simulink model "MotorCtrl_DTC_Math"  (R2023b)
settings: Solver=FixedStepDiscrete  StartTime=0.0  StopTime=5  FixedStep=MC_Sim_BaseStep  RelTol=1e-3  EnableMultiTasking=on
values from neighbouring files (symbols this model uses):
  MC_ADC_BitNum = 0.0    [MotorControlDataDictionary_Math.sldd]
  MC_ADC_Offset = 0.0    [MotorControlDataDictionary_Math.sldd]
  MC_ADC_VRef = 1.0    [MotorControlDataDictionary_Math.sldd]
  MC_Const_DutyL = 0.2    [MotorControlDataDictionary_Math.sldd]
  MC_Const_DutyS = 0.8    [MotorControlDataDictionary_Math.sldd]
  MC_CSA_Gain = 1.0    [MotorControlDataDictionary_Math.sldd]
  MC_Input_Vdc = 13.5    [MotorControlDataDictionary_Math.sldd]
  MC_MOS_DeadTime = 1.0E-6    [MotorControlDataDictionary_Math.sldd]
  MC_Motor_Mechinal_Damp = 1.0E-5    [MotorControlDataDictionary_Math.sldd]
  MC_Motor_Mechinal_Fric = 0.0    [MotorControlDataDictionary_Math.sldd]
  MC_Motor_Mechinal_Inertia = 0.0103    [MotorControlDataDictionary_Math.sldd]
  MC_Motor_Phi = 0.0059190254913385806    [MotorControlDataDictionary_Math.sldd]
  MC_Motor_Rotor_Pn = 4.0    [MotorControlDataDictionary_Math.sldd]
  MC_Motor_Stator_Ld = 5.6345E-5    [MotorControlDataDictionary_Math.sldd]
  MC_Motor_Stator_Lq = 5.6345E-5    [MotorControlDataDictionary_Math.sldd]
  MC_Motor_Stator_Rs = 0.0286    [MotorControlDataDictionary_Math.sldd]
  MC_Param_CurrentPI_Ki = 0.0071879639914134473    [MotorControlDataDictionary_Math.sldd]
  MC_Param_CurrentPI_Kp = 0.283220860906427    [MotorControlDataDictionary_Math.sldd]
  MC_Param_CurrentPI_UdInteMax = 7.794228634059948    [MotorControlDataDictionary_Math.sldd]
  MC_Param_CurrentPI_UdInteMin = -7.794228634059948    [MotorControlDataDictionary_Math.sldd]
  MC_Param_CurrentPI_UdMax = 7.794228634059948    [MotorControlDataDictionary_Math.sldd]
  MC_Param_CurrentPI_UdMin = -7.794228634059948    [MotorControlDataDictionary_Math.sldd]
  MC_Param_CurrentPI_UqInteMax = 7.794228634059948    [MotorControlDataDictionary_Math.sldd]
  MC_Param_CurrentPI_UqInteMin = -7.794228634059948    [MotorControlDataDictionary_Math.sldd]
  MC_Param_CurrentPI_UqMax = 7.794228634059948    [MotorControlDataDictionary_Math.sldd]
  MC_Param_CurrentPI_UqMin = -7.794228634059948    [MotorControlDataDictionary_Math.sldd]
  MC_Param_Flux_Gamma = 750000.0    [MotorControlDataDictionary_Math.sldd]
  MC_Param_Flux_Lalpha = 5.6345E-5    [MotorControlDataDictionary_Math.sldd]
  MC_Param_Flux_Lbeta = 5.6345E-5    [MotorControlDataDictionary_Math.sldd]
  MC_Param_Flux_Ralpha = 0.0286    [MotorControlDataDictionary_Math.sldd]
  MC_Param_Flux_Rbeta = 0.0286    [MotorControlDataDictionary_Math.sldd]
  MC_Param_Luen_BEMFalpha = -17747.803709290976    [MotorControlDataDictionary_Math.sldd]
  MC_Param_Luen_BEMFbeta = -17747.803709290976    [MotorControlDataDictionary_Math.sldd]
  MC_Param_Luen_BEMFErr = -8.0    [MotorControlDataDictionary_Math.sldd]
  MC_Param_Luen_Currentalpha = -507.58718608572195    [MotorControlDataDictionary_Math.sldd]
  MC_Param_Luen_Currentbeta = -507.58718608572195    [MotorControlDataDictionary_Math.sldd]
  MC_Param_Luen_CurrentErr = -8.0    [MotorControlDataDictionary_Math.sldd]
  MC_Param_Luen_PLL_Ki = 2.3480975196640594    [MotorControlDataDictionary_Math.sldd]
  MC_Param_Luen_PLL_Kp = 153.24842212633141    [MotorControlDataDictionary_Math.sldd]
  MC_Param_Luen_Voltagealpha = 17747.803709290976    [MotorControlDataDictionary_Math.sldd]
  MC_Param_Luen_Voltagebeta = 17747.803709290976    [MotorControlDataDictionary_Math.sldd]
  MC_Param_PhasetoReal = 500.0    [MotorControlDataDictionary_Math.sldd]
  MC_Param_SMO_CoffA = 0.97462064069571386    [MotorControlDataDictionary_Math.sldd]
  MC_Param_SMO_CoffB = 0.88739018546454884    [MotorControlDataDictionary_Math.sldd]
  MC_Param_SpeedCtrl_IdMax = 60.0    [MotorControlDataDictionary_Math.sldd]
  MC_Param_SpeedCtrl_IdMin = -60.0    [MotorControlDataDictionary_Math.sldd]
  MC_Param_SpeedCtrl_IqMax = 60.0    [MotorControlDataDictionary_Math.sldd]
  MC_Param_SpeedCtrl_IqMin = -60.0    [MotorControlDataDictionary_Math.sldd]
  MC_Param_SpeedPI_Ki = 0.57248683633241571    [MotorControlDataDictionary_Math.sldd]
  MC_Param_SpeedPI_Kp = 9.1114109857344836    [MotorControlDataDictionary_Math.sldd]
  MC_Param_SpeedtoTheta = 5.0E-5    [MotorControlDataDictionary_Math.sldd]
  MC_Param_SVPWM_DutyMax = 0.98    [MotorControlDataDictionary_Math.sldd]
  MC_Param_SVPWM_DutyMin = 0.02    [MotorControlDataDictionary_Math.sldd]
  MC_Param_SVPWM_SampleOffset1 = 0.02    [MotorControlDataDictionary_Math.sldd]
  MC_Param_SVPWM_SampleOffset2 = 0.015    [MotorControlDataDictionary_Math.sldd]
  MC_Param_SVPWM_SampleValid = 0.011999999999999999    [MotorControlDataDictionary_Math.sldd]
  MC_Sample_CurrentNoise = 1.0E-15    [MotorControlDataDictionary_Math.sldd]
  MC_Sample_Rs = 0.002    [MotorControlDataDictionary_Math.sldd]
  MC_Sample_VbusNoise = 1.0E-15    [MotorControlDataDictionary_Math.sldd]
  MC_Sim_BaseStep = 5.0E-8    [MotorControlDataDictionary_Math.sldd]
  MC_Sim_HFTStep = 5.0E-5    [MotorControlDataDictionary_Math.sldd]
  MC_Sim_MFTStep = 0.002    [MotorControlDataDictionary_Math.sldd]
libraries: simulink x29, spsVoltageMeasurementLib x2, spsDCVoltageSourceLib x1, spsGroundLib x1, spsPermanentMagnetSynchronousMachineLib x1, spsSeriesRLCBranchLib x1, spsThreePhaseVIMeasurementLib x1, spsUniversalBridgeLib x1, sps_lib x1
(part 2 of 5)

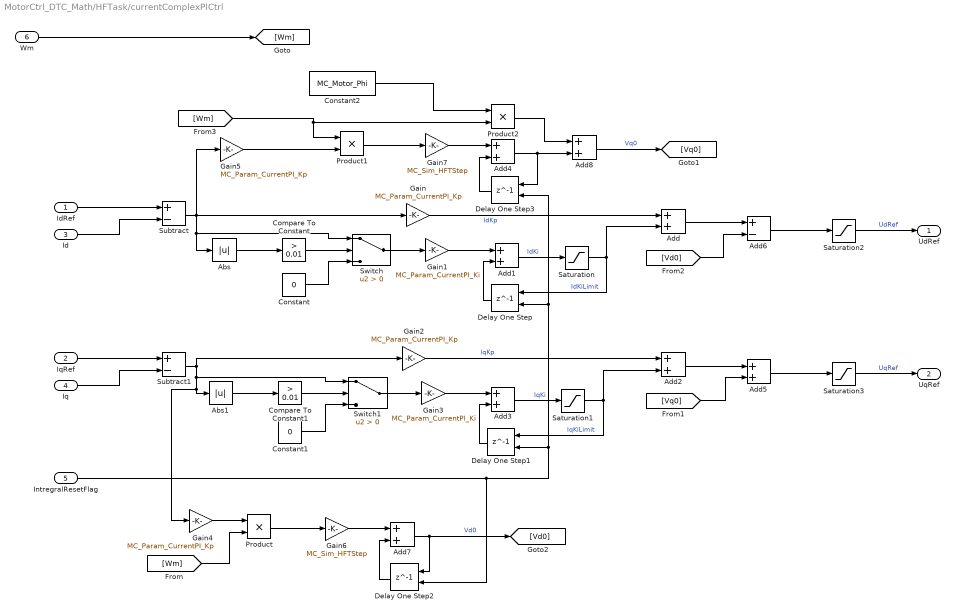
== system MotorCtrl_DTC_Math/HFTask/currentComplexPICtrl ==
  IdRef : Inport
  IqRef : Inport  Port=2
  Id : Inport  Port=3
  Iq : Inport  Port=4
  IntregralResetFlag : Inport  Port=5
  Wm : Inport  Port=6
  Abs : Abs  SaturateOnIntegerOverflow=off
  Abs1 : Abs  SaturateOnIntegerOverflow=off
  Add{,2,5,8} (4 alike) : Sum
  Add{1,3..4,7} (4 alike) : Sum  OutDataTypeStr=single
  Add6 : Sum  Inputs=+-
  Compare To Constant : simulink/Logic and Bit Operations/Compare To Constant  relop=>  const=0.01  OutDataTypeStr=boolean
  Compare To Constant1 : simulink/Logic and Bit Operations/Compare To Constant  relop=>  const=0.01  OutDataTypeStr=boolean
  Constant : Constant  Value=0  OutDataTypeStr=single
  Constant1 : Constant  Value=0  OutDataTypeStr=single
  Constant2 : Constant  Value=MC_Motor_Phi  OutDataTypeStr=single
  Delay One Step{,1..3} (4 alike) : Delay  DelayLength=1  ExternalReset=Level
      settings: InputPortMap=u0,r5
  Gain : Gain  Gain=MC_Param_CurrentPI_Kp  OutDataTypeStr=single
  Gain1 : Gain  Gain=MC_Param_CurrentPI_Ki  OutDataTypeStr=single
  Gain2 : Gain  Gain=MC_Param_CurrentPI_Kp  OutDataTypeStr=single
  Gain3 : Gain  Gain=MC_Param_CurrentPI_Ki  OutDataTypeStr=single
  Gain4 : Gain  Gain=MC_Param_CurrentPI_Kp
  Gain5 : Gain  Gain=MC_Param_CurrentPI_Kp
  Gain6 : Gain  Gain=MC_Sim_HFTStep  OutDataTypeStr=single
  Gain7 : Gain  Gain=MC_Sim_HFTStep  OutDataTypeStr=single
  Product : Product
  Product1 : Product
  Product2 : Product
  Saturation : Saturate  UpperLimit=MC_Param_CurrentPI_UdInteMax  LowerLimit=MC_Param_CurrentPI_UdInteMin
  Saturation1 : Saturate  UpperLimit=MC_Param_CurrentPI_UqInteMax  LowerLimit=MC_Param_CurrentPI_UqInteMin
  Saturation2 : Saturate  UpperLimit=MC_Param_CurrentPI_UdMax  LowerLimit=MC_Param_CurrentPI_UdMin
  Saturation3 : Saturate  UpperLimit=MC_Param_CurrentPI_UqMax  LowerLimit=MC_Param_CurrentPI_UqMin
  Subtract : Sum  Inputs=+-
  Subtract1 : Sum  Inputs=+-
  Switch : Switch  Criteria=u2 > Threshold  SaturateOnIntegerOverflow=off  InputSameDT=off
  Switch1 : Switch  Criteria=u2 > Threshold  SaturateOnIntegerOverflow=off  InputSameDT=off
  UdRef : Outport
  UqRef : Outport  Port=2
  wires:
  Wm/1 -> [Wm]
  Saturation3/1 -> UqRef/1  "UqRef"
  Saturation2/1 -> UdRef/1  "UdRef"
  [Vd0] -> Add6/2
  Add6/1 -> Saturation2/1
  Add/1 -> Add6/1
  [Vq0] -> Add5/2
  Add2/1 -> Add5/1
  [Wm] -> Product/2
  Id/1 -> Subtract/2
  Gain4/1 -> Product/1
  Switch1/1 -> Gain3/1
  Abs1/1 -> Compare To Constant1/1
  Compare To Constant1/1 -> Switch1/2
  Constant1/1 -> Switch1/3
  Constant/1 -> Switch/3
  Compare To Constant/1 -> Switch/2
  Switch/1 -> Gain1/1
  Add5/1 -> Saturation3/1
  IqRef/1 -> Subtract1/1
  Iq/1 -> Subtract1/2
  Subtract1/1 -> Gain2/1, Gain4/1, Abs1/1, Switch1/1
  Gain2/1 -> Add2/1  "IqKp"
  Gain3/1 -> Add3/1
  Delay One Step1/1 -> Add3/2
  Add3/1 -> Saturation1/1  "IqKi"
  Saturation1/1 -> Add2/2, Delay One Step1/1  "IqKiLimit"
  Saturation/1 -> Delay One Step/1, Add/2  "IdKiLimit"
  Add1/1 -> Saturation/1  "IdKi"
  Delay One Step/1 -> Add1/2
  Gain1/1 -> Add1/1
  Abs/1 -> Compare To Constant/1
  Gain/1 -> Add/1  "IdKp"
  Subtract/1 -> Gain5/1, Abs/1, Switch/1, Gain/1
  IdRef/1 -> Subtract/1
  Gain6/1 -> Add7/1
  Product/1 -> Gain6/1
  Delay One Step2/1 -> Add7/2
  Add7/1 -> [Vd0], Delay One Step2/1  "Vd0"
  Add4/1 -> Delay One Step3/1, Add8/2
  Delay One Step3/1 -> Add4/2
  Gain7/1 -> Add4/1
  IntregralResetFlag/1 -> Delay One Step2/2, Delay One Step1/2, Delay One Step3/2, Delay One Step/2
  Product1/1 -> Gain7/1
  Constant2/1 -> Product2/1
  Gain5/1 -> Product1/2
  Add8/1 -> [Vq0]  "Vq0"
  Product2/1 -> Add8/1
  [Wm] -> Product1/1, Product2/2

== system MotorCtrl_DTC_Math/HFTask/currentDBC ==
  note: 无差拍电流控制器（延时1拍）
  IdRef : Inport
  IqRef : Inport  Port=2
  Id : Inport  Port=3
  Iq : Inport  Port=4
  Wm : Inport  Port=5
  Add5 : Sum  Inputs=++-
  Add6 : Sum  Inputs=+++
  Add7 : Sum
  Constant1 : Constant  Value=MC_Motor_Phi  OutDataTypeStr=single
  Gain10 : Gain  Gain=MC_Motor_Stator_Lq
  Gain11 : Gain  Gain=MC_Motor_Stator_Lq/MC_Sim_HFTStep
  Gain12 : Gain  Gain=MC_Motor_Stator_Rs-(MC_Motor_Stator_Lq/MC_Sim_HFTStep)
  Gain13 : Gain  Gain=MC_Motor_Stator_Ld
  Gain8 : Gain  Gain=MC_Motor_Stator_Ld/MC_Sim_HFTStep
  Gain9 : Gain  Gain=MC_Motor_Stator_Rs-(MC_Motor_Stator_Ld/MC_Sim_HFTStep)
  Product2 : Product
  Product3 : Product
  Saturation : Saturate  UpperLimit=MC_Param_CurrentPI_UdMax  LowerLimit=MC_Param_CurrentPI_UdMin
  Saturation1 : Saturate  UpperLimit=MC_Param_CurrentPI_UqMax  LowerLimit=MC_Param_CurrentPI_UqMin
  UdRef : Outport
  UqRef : Outport  Port=2
  wires:
  Wm/1 -> [Wm]
  Iq/1 -> [Iq]
  Id/1 -> [Id]
  IqRef/1 -> [IqRef]
  IdRef/1 -> [IdRef]
  [IdRef] -> Gain8/1
  Gain8/1 -> Add5/1  "IdRef_Vd"
  [Id] -> Gain9/1
  Gain9/1 -> Add5/2  "Id_Vd"
  [Iq] -> Gain10/1
  Gain10/1 -> Product2/2
  [Wm] -> Product2/1
  [IqRef] -> Gain11/1
  Gain11/1 -> Add6/1  "IqRef_Vq"
  Gain12/1 -> Add6/2  "Iq_Vq"
  [Iq] -> Gain12/1
  [Wm] -> Product3/1
  Add7/1 -> Product3/2
  Constant1/1 -> Add7/2
  Gain13/1 -> Add7/1
  [Id] -> Gain13/1
  Saturation/1 -> UdRef/1  "UdRef_DBC"
  Saturation1/1 -> UqRef/1  "UqRef_DBC"
  Add5/1 -> Saturation/1
  Product2/1 -> Add5/3  "Iq_Vd"
  Add6/1 -> Saturation1/1
  Product3/1 -> Add6/3  "Id_Vq"

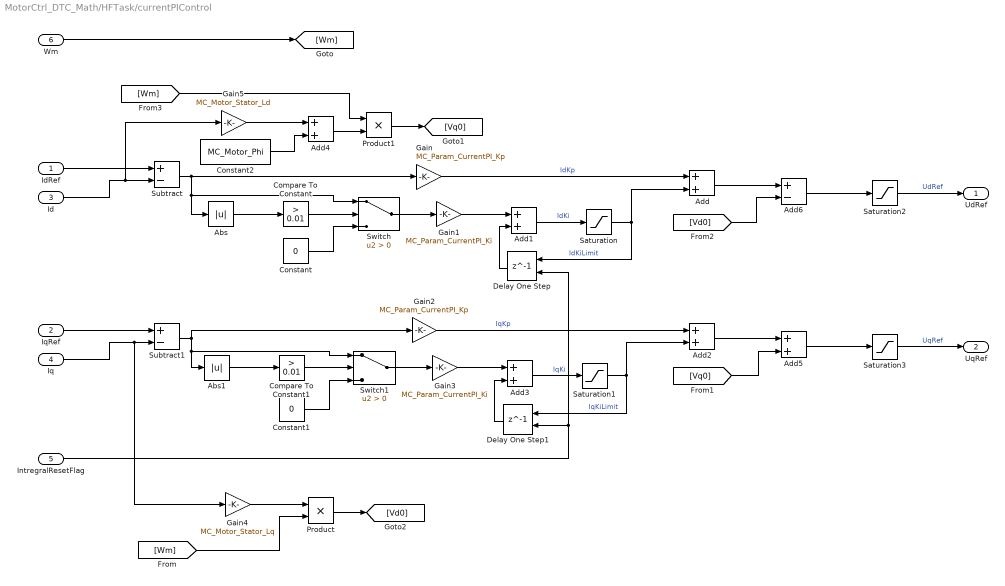
== system MotorCtrl_DTC_Math/HFTask/currentPIControl ==
  IdRef : Inport
  IqRef : Inport  Port=2
  Id : Inport  Port=3
  Iq : Inport  Port=4
  IntregralResetFlag : Inport  Port=5
  Wm : Inport  Port=6
  Abs : Abs  SaturateOnIntegerOverflow=off
  Abs1 : Abs  SaturateOnIntegerOverflow=off
  Add{,2,4..5} (4 alike) : Sum
  Add1 : Sum  OutDataTypeStr=single
  Add3 : Sum  OutDataTypeStr=single
  Add6 : Sum  Inputs=+-
  Compare To Constant : simulink/Logic and Bit Operations/Compare To Constant  relop=>  const=0.01  OutDataTypeStr=boolean
  Compare To Constant1 : simulink/Logic and Bit Operations/Compare To Constant  relop=>  const=0.01  OutDataTypeStr=boolean
  Constant : Constant  Value=0  OutDataTypeStr=single
  Constant1 : Constant  Value=0  OutDataTypeStr=single
  Constant2 : Constant  Value=MC_Motor_Phi  OutDataTypeStr=single
  Delay One Step : Delay  DelayLength=1  ExternalReset=Level
      settings: InputPortMap=u0,r5
  Delay One Step1 : Delay  DelayLength=1  ExternalReset=Level
      settings: InputPortMap=u0,r5
  Gain : Gain  Gain=MC_Param_CurrentPI_Kp  OutDataTypeStr=single
  Gain1 : Gain  Gain=MC_Param_CurrentPI_Ki  OutDataTypeStr=single
  Gain2 : Gain  Gain=MC_Param_CurrentPI_Kp  OutDataTypeStr=single
  Gain3 : Gain  Gain=MC_Param_CurrentPI_Ki  OutDataTypeStr=single
  Gain4 : Gain  Gain=MC_Motor_Stator_Lq
  Gain5 : Gain  Gain=MC_Motor_Stator_Ld
  Product : Product
  Product1 : Product
  Saturation : Saturate  UpperLimit=MC_Param_CurrentPI_UdInteMax  LowerLimit=MC_Param_CurrentPI_UdInteMin
  Saturation1 : Saturate  UpperLimit=MC_Param_CurrentPI_UqInteMax  LowerLimit=MC_Param_CurrentPI_UqInteMin
  Saturation2 : Saturate  UpperLimit=MC_Param_CurrentPI_UdMax  LowerLimit=MC_Param_CurrentPI_UdMin
  Saturation3 : Saturate  UpperLimit=MC_Param_CurrentPI_UqMax  LowerLimit=MC_Param_CurrentPI_UqMin
  Subtract : Sum  Inputs=+-
  Subtract1 : Sum  Inputs=+-
  Switch : Switch  Criteria=u2 > Threshold  SaturateOnIntegerOverflow=off  InputSameDT=off
  Switch1 : Switch  Criteria=u2 > Threshold  SaturateOnIntegerOverflow=off  InputSameDT=off
  UdRef : Outport
  UqRef : Outport  Port=2
  wires:
  IdRef/1 -> Subtract/1
  Subtract/1 -> Gain/1, Switch/1, Abs/1
  Gain/1 -> Add/1  "IdKp"
  Abs/1 -> Compare To Constant/1
  Gain1/1 -> Add1/1
  Delay One Step/1 -> Add1/2
  Add1/1 -> Saturation/1  "IdKi"
  Saturation/1 -> Add/2, Delay One Step/1  "IdKiLimit"
  Saturation1/1 -> Delay One Step1/1, Add2/2  "IqKiLimit"
  Add3/1 -> Saturation1/1  "IqKi"
  Delay One Step1/1 -> Add3/2
  Gain3/1 -> Add3/1
  Gain2/1 -> Add2/1  "IqKp"
  Subtract1/1 -> Switch1/1, Abs1/1, Gain2/1
  Iq/1 -> Gain4/1, Subtract1/2
  IqRef/1 -> Subtract1/1
  IntregralResetFlag/1 -> Delay One Step/2, Delay One Step1/2
  Add5/1 -> Saturation3/1
  Switch/1 -> Gain1/1
  Compare To Constant/1 -> Switch/2
  Constant/1 -> Switch/3
  Constant1/1 -> Switch1/3
  Compare To Constant1/1 -> Switch1/2
  Abs1/1 -> Compare To Constant1/1
  Switch1/1 -> Gain3/1
  Gain4/1 -> Product/1
  Id/1 -> Gain5/1, Subtract/2
  [Wm] -> Product/2
  Gain5/1 -> Add4/1
  Add4/1 -> Product1/2
  Constant2/1 -> Add4/2
  Product1/1 -> [Vq0]
  Product/1 -> [Vd0]
  Add2/1 -> Add5/1
  [Vq0] -> Add5/2
  Add/1 -> Add6/1
  Add6/1 -> Saturation2/1
  [Vd0] -> Add6/2
  Saturation2/1 -> UdRef/1  "UdRef"
  Saturation3/1 -> UqRef/1  "UqRef"
  [Wm] -> Product1/1
  Wm/1 -> [Wm]

== system MotorCtrl_DTC_Math/HFTask/fluxobservor ==
  Valpha : Inport
  Vbeta : Inport  Port=2
  Ialpha : Inport  Port=3
  Ibeta : Inport  Port=4
  getFlux : Subsystem
  getSpeedandTheta : Subsystem
  Speed : Outport
  Theta : Outport  Port=2
  wires:
  getSpeedandTheta/2(Theta) -> Theta/1
  getSpeedandTheta/1(Speed) -> Speed/1
  getFlux/2(Phibeta) -> getSpeedandTheta/2(Phibeta)
  getFlux/1(Phialpha) -> getSpeedandTheta/1(Phialpha)
  Ibeta/1 -> getFlux/4(Ibeta)
  Ialpha/1 -> getFlux/3(Ialpha)
  Vbeta/1 -> getFlux/2(Vbeta)
  Valpha/1 -> getFlux/1(Valpha)

== system MotorCtrl_DTC_Math/HFTask/getCurrentPredict ==
  note: 开发日志：
      | 2025.03.26:
      | 1、完成两节拍的电流预测
      | 2025.03.27：
      | 1、采用延时2个周期的采样电流和延时1个周期的设定电压进行延时1个周期的电机电流预测
  Ud1 : Inport
  Id : Inport  Port=2
  Uq1 : Inport  Port=3
  Iq : Inport  Port=4
  Wm : Inport  Port=5
  Add : Sum  Inputs=+++
  Add1 : Sum  Inputs=++-
  Add2 : Sum
  Constant : Constant  Value=MC_Motor_Phi  OutDataTypeStr=single
  Gain1 : Gain  Gain=MC_Sim_HFTStep/MC_Motor_Stator_Lq
  Gain4 : Gain  Gain=MC_Sim_HFTStep/MC_Motor_Stator_Ld
  Gain5 : Gain  Gain=1-(MC_Sim_HFTStep*MC_Motor_Stator_Rs/MC_Motor_Stator_Ld)
  Gain6 : Gain  Gain=MC_Sim_HFTStep/MC_Motor_Stator_Lq
  Gain7 : Gain  Gain=1-(MC_Sim_HFTStep*MC_Motor_Stator_Rs/MC_Motor_Stator_Lq)
  Gain8 : Gain  Gain=MC_Sim_HFTStep*MC_Motor_Stator_Ld/MC_Motor_Stator_Lq
  Gain9 : Gain  Gain=(MC_Sim_HFTStep*MC_Motor_Stator_Lq/MC_Motor_Stator_Ld)
  Product : Product
  Product1 : Product
  Id_Pre : Outport
  Iq_Pre : Outport  Port=2
  wires:
  [Iq] -> Gain7/1
  [Wm] -> Product1/1
  Iq/1 -> [Iq]
  Gain4/1 -> Add/1  "Ud_Id1"
  [Iq] -> Gain9/1
  [Uq1] -> Gain6/1
  Gain9/1 -> Product/1
  Constant/1 -> Gain1/1
  Product/1 -> Add/3  "Iq_Id1"
  [Ud1] -> Gain4/1
  Gain6/1 -> Add1/1  "Uq_Iq1"
  Gain7/1 -> Add1/2  "Iq_Iq1"
  Gain5/1 -> Add/2  "Id_Id1"
  [Id] -> Gain8/1
  Product1/1 -> Add1/3  "Id_Iq1"
  Gain8/1 -> Add2/1
  [Wm] -> Product/2
  Id/1 -> [Id]
  Add2/1 -> Product1/2
  [Id] -> Gain5/1
  Wm/1 -> [Wm]
  Gain1/1 -> Add2/2
  Add/1 -> Id_Pre/1  "Id1"
  Add1/1 -> Iq_Pre/1  "Iq1"
  Ud1/1 -> [Ud1]
  Uq1/1 -> [Uq1]

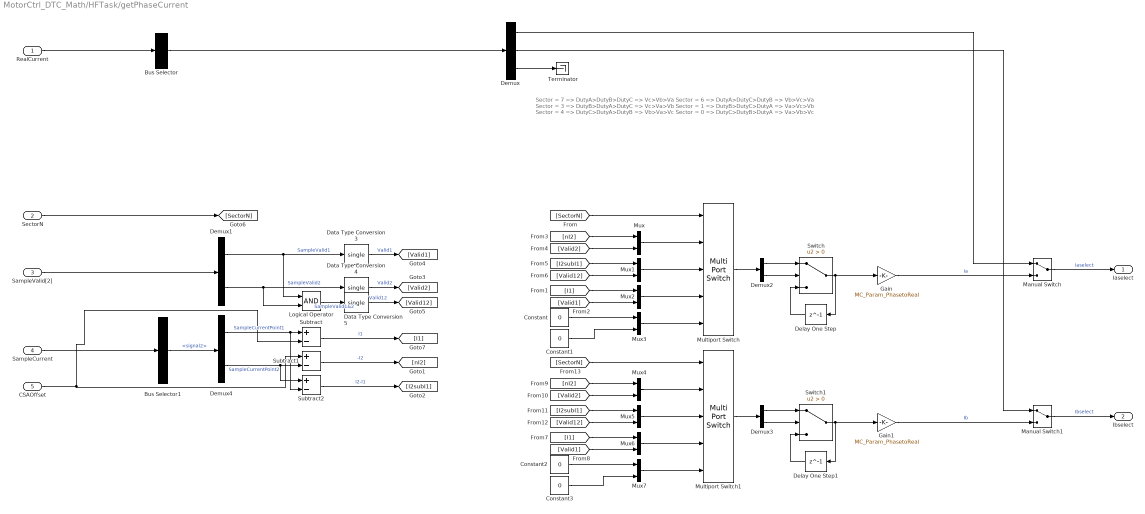
== system MotorCtrl_DTC_Math/HFTask/getPhaseCurrent ==
  note: Sector = 7 => DutyA>DutyB>DutyC => Vc>Vb>Va
      | Sector = 6 => DutyA>DutyC>DutyB => Vb>Vc>Va
      | Sector = 3 => DutyB>DutyA>DutyC => Vc>Va>Vb
      | Sector = 1 => DutyB>DutyC>DutyA => Va>Vc>Vb
      | Sector = 4 => DutyC>DutyA>DutyB => Vb>Va>Vc
      | Sector = 0 => DutyC>DutyB>DutyA => Va>Vb>Vc
  RealCurrent : Inport
  SectorN : Inport  Port=2
  SampleValid[2] : Inport  Port=3
  SampleCurrent : Inport  Port=4
  CSAOffset : Inport  Port=5
  Bus Selector : BusSelector  OutputSignals=PhaseI  OutputAsBus=on
  Bus Selector1 : BusSelector  OutputSignals=signal2
  Constant{,1..3} (4 alike) : Constant  Value=0  OutDataTypeStr=single
  Data Type Conversion3 : DataTypeConversion  OutDataTypeStr=single  RndMeth=Simplest  SaturateOnIntegerOverflow=off
  Data Type Conversion4 : DataTypeConversion  OutDataTypeStr=single  RndMeth=Simplest  SaturateOnIntegerOverflow=off
  Data Type Conversion5 : DataTypeConversion  OutDataTypeStr=single  RndMeth=Simplest  SaturateOnIntegerOverflow=off
  Delay One Step : Delay  DelayLength=1
  Delay One Step1 : Delay  DelayLength=1
  Demux : Demux  Outputs=3
  Demux{1..4} (4 alike) : Demux  Outputs=2
  Gain : Gain  Gain=MC_Param_PhasetoReal
  Gain1 : Gain  Gain=MC_Param_PhasetoReal
  Logical Operator : Logic  AllPortsSameDT=off  OutDataTypeStr=boolean
  Manual Switch : ManualSwitch
  Manual Switch1 : ManualSwitch
  Multiport Switch : MultiPortSwitch  DataPortOrder=Specify indices  DataPortIndices={[7,6],[3,4],[0,1]}  DataPortForDefault=Additional data port  SaturateOnIntegerOverflow=off  InputSameDT=off
  Multiport Switch1 : MultiPortSwitch  DataPortOrder=Specify indices  DataPortIndices={[3,1],[7,0],[6,4]}  DataPortForDefault=Additional data port  SaturateOnIntegerOverflow=off  InputSameDT=off
  Mux{,1..7} (8 alike) : Mux  Inputs=2
  Subtract : Sum  Inputs=+-
  Subtract1 : Sum  Inputs=+-
  Subtract2 : Sum  Inputs=+-
  Switch : Switch  Criteria=u2 > Threshold  SaturateOnIntegerOverflow=off  InputSameDT=off
  Switch1 : Switch  Criteria=u2 > Threshold  SaturateOnIntegerOverflow=off  InputSameDT=off
  Terminator : Terminator
  Iaselect : Outport
  Ibselect : Outport  Port=2
  wires:
  RealCurrent/1 -> Bus Selector/1
  Bus Selector/1 -> Demux/1
  Manual Switch/1 -> Iaselect/1  "Iaselect"
  Demux/3 -> Terminator/1
  Manual Switch1/1 -> Ibselect/1  "Ibselect"
  Multiport Switch1/1 -> Demux3/1
  Demux3/2 -> Switch1/2
  Demux3/1 -> Switch1/1
  Switch1/1 -> Delay One Step1/1, Gain1/1
  Delay One Step1/1 -> Switch1/3
  Gain1/1 -> Manual Switch1/2  "Ib"
  Gain/1 -> Manual Switch/2  "Ia"
  Delay One Step/1 -> Switch/3
  Switch/1 -> Gain/1, Delay One Step/1
  Demux2/1 -> Switch/1
  Demux2/2 -> Switch/2
  Multiport Switch/1 -> Demux2/1
  [SectorN] -> Multiport Switch1/1
  Mux4/1 -> Multiport Switch1/2
  Mux5/1 -> Multiport Switch1/3
  Mux6/1 -> Multiport Switch1/4
  [I1] -> Mux6/1
  [Valid1] -> Mux6/2
  [nI2] -> Mux4/1
  [Valid2] -> Mux4/2
  [Valid12] -> Mux5/2
  [I2subI1] -> Mux5/1
  Mux7/1 -> Multiport Switch1/5
  Constant2/1 -> Mux7/1
  Constant3/1 -> Mux7/2
  Subtract/1 -> [I1]  "I1"
  Subtract1/1 -> [nI2]  "-I2"
  Data Type Conversion5/1 -> [Valid12]  "Valid12"
  Data Type Conversion4/1 -> [Valid2]  "Valid2"
  Data Type Conversion3/1 -> [Valid1]  "Valid1"
  Subtract2/1 -> [I2subI1]  "I2-I1"
  Constant1/1 -> Mux3/2
  Constant/1 -> Mux3/1
  Mux3/1 -> Multiport Switch/5
  [I2subI1] -> Mux1/1
  [Valid12] -> Mux1/2
  [Valid2] -> Mux/2
  [nI2] -> Mux/1
  [Valid1] -> Mux2/2
  [I1] -> Mux2/1
  [SectorN] -> Multiport Switch/1
  SectorN/1 -> [SectorN]
  Mux2/1 -> Multiport Switch/4
  Mux1/1 -> Multiport Switch/3
  Mux/1 -> Multiport Switch/2
  Logical Operator/1 -> Data Type Conversion5/1  "SampleValid1&2"
  Demux1/2 -> Data Type Conversion4/1, Logical Operator/2  "SampleValid2"
  Demux1/1 -> Data Type Conversion3/1, Logical Operator/1  "SampleValid1"
  SampleValid[2]/1 -> Demux1/1
  Demux4/2 -> Subtract2/1, Subtract1/2  "SampleCurrentPoint2"
  CSAOffset/1 -> Subtract1/1, Subtract/2
  Demux4/1 -> Subtract2/2, Subtract/1  "SampleCurrentPoint1"
  Bus Selector1/1 -> Demux4/1  "<signal2>"
  SampleCurrent/1 -> Bus Selector1/1
  Demux/1 -> Manual Switch/1
  Demux/2 -> Manual Switch1/1

== system MotorCtrl_DTC_Math/HFTask/getSinCos ==
  Theta : Inport
  Sin : Trigonometry
  Sin1 : Trigonometry  Operator=cos
  SinTheta : Outport
  CosTheta : Outport  Port=2
  wires:
  Theta/1 -> Sin1/1, Sin/1
  Sin/1 -> SinTheta/1
  Sin1/1 -> CosTheta/1

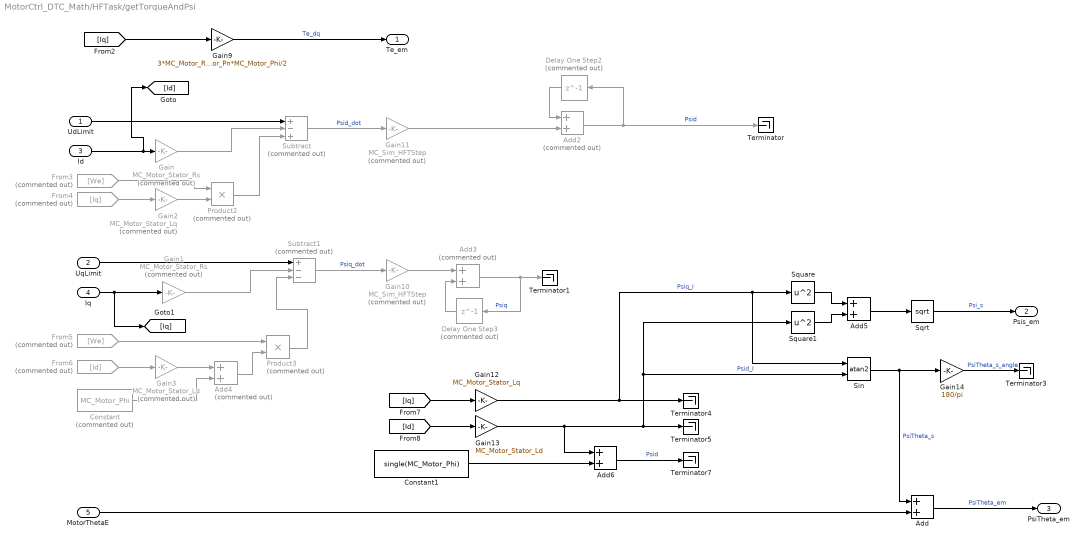
== system MotorCtrl_DTC_Math/HFTask/getTorqueAndPsi ==
  UdLimit : Inport
  UqLimit : Inport  Port=2
  Id : Inport  Port=3
  Iq : Inport  Port=4
  "MotorThetaE " : Inport  Port=5
  Add : Sum
  Add2 : Sum  Commented=on
  Add3 : Sum  Commented=on
  Add4 : Sum  Commented=on
  Add5 : Sum
  Add6 : Sum
  Constant : Constant  Commented=on  Value=MC_Motor_Phi
  Constant1 : Constant  Value=single(MC_Motor_Phi)
  Delay One Step2 : Delay  Commented=on  DelayLength=1
  Delay One Step3 : Delay  Commented=on  DelayLength=1
  From3 : From  Commented=on  GotoTag=We
  From4 : From  Commented=on  GotoTag=Iq
  From5 : From  Commented=on  GotoTag=We
  From6 : From  Commented=on  GotoTag=Id
  Gain : Gain  Commented=on  Gain=MC_Motor_Stator_Rs
  Gain1 : Gain  Commented=on  Gain=MC_Motor_Stator_Rs
  Gain10 : Gain  Commented=on  Gain=MC_Sim_HFTStep
  Gain11 : Gain  Commented=on  Gain=MC_Sim_HFTStep
  Gain12 : Gain  Gain=MC_Motor_Stator_Lq  OutDataTypeStr=single  RndMeth=Simplest
  Gain13 : Gain  Gain=MC_Motor_Stator_Ld  OutDataTypeStr=single  RndMeth=Simplest
  Gain14 : Gain  Gain=180/pi
  Gain2 : Gain  Commented=on  Gain=MC_Motor_Stator_Lq
  Gain3 : Gain  Commented=on  Gain=MC_Motor_Stator_Ld
  Gain9 : Gain  Gain=3*MC_Motor_Rotor_Pn*MC_Motor_Phi/2
  Product2 : Product  Commented=on
  Product3 : Product  Commented=on
  Sin : Trigonometry  Operator=atan2
  Sqrt : Sqrt
  Square : Math  Operator=square
  Square1 : Math  Operator=square
  Subtract : Sum  Commented=on  Inputs=+-+
  Subtract1 : Sum  Commented=on  Inputs=+--
  Terminator{,1,3..5,7} (6 alike) : Terminator
  Te_em : Outport
  Psis_em : Outport  Port=2
  PsiTheta_em : Outport  Port=3
  wires:
  UdLimit/1 -> Subtract/1
  Id/1 -> [Id], Gain/1
  Gain/1 -> Subtract/2
  UqLimit/1 -> Subtract1/1
  Gain1/1 -> Subtract1/2
  Iq/1 -> [Iq], Gain1/1
  [Iq] -> Gain9/1
  Gain9/1 -> Te_em/1  "Te_dq"
  Add2/1 -> Delay One Step2/1, Terminator/1  "Psid"
  Delay One Step3/1 -> Add3/2
  Add3/1 -> Delay One Step3/1, Terminator1/1  "Psiq"
  Delay One Step2/1 -> Add2/1
  From4/1 -> Gain2/1
  Subtract1/1 -> Gain10/1  "Psiq_dot"
  Gain2/1 -> Product2/2
  From3/1 -> Product2/1
  Product2/1 -> Subtract/3
  Subtract/1 -> Gain11/1  "Psid_dot"
  From6/1 -> Gain3/1
  From5/1 -> Product3/1
  Add4/1 -> Product3/2
  Product3/1 -> Subtract1/3
  Gain3/1 -> Add4/1
  Constant/1 -> Add4/2
  Gain10/1 -> Add3/1
  Gain11/1 -> Add2/2
  [Iq] -> Gain12/1
  [Id] -> Gain13/1
  Constant1/1 -> Add6/2
  Gain12/1 -> Sin/1, Square/1, Terminator4/1  "Psiq_I"
  Gain13/1 -> Add6/1, Sin/2, Square1/1, Terminator5/1  "Psid_I"
  Square/1 -> Add5/1
  Square1/1 -> Add5/2
  Add5/1 -> Sqrt/1
  Sqrt/1 -> Psis_em/1  "Psi_s"
  Add6/1 -> Terminator7/1  "Psid"
  Sin/1 -> Add/1, Gain14/1  "PsiTheta_s"
  Gain14/1 -> Terminator3/1  "PsiTheta_s_angle"
  Add/1 -> PsiTheta_em/1  "PsiTheta_em"
  "MotorThetaE "/1 -> Add/2

== system MotorCtrl_DTC_Math/HFTask/getVdq ==
  TeRef : Inport
  TeEm : Inport  Port=2
  PsiRef : Inport  Port=3
  PsiEm : Inport  Port=4
  Add1 : Sum
  Add2 : Sum
  Delay One Step14 : Delay  DelayLength=1
  Gain7 : Gain  Gain=0.1
  Gain8 : Gain  Gain=0.1*MC_Sim_HFTStep
  Subtract : Sum  Inputs=+-
  Subtract1 : Sum  Inputs=+-
  Out1 : Outport
  wires:
  Gain7/1 -> Add2/1
  Add1/1 -> Add2/2, Delay One Step14/1
  Delay One Step14/1 -> Add1/2
  Add2/1 -> ?  "ThetaTe"
  Gain8/1 -> Add1/1
  TeRef/1 -> Subtract/1
  TeEm/1 -> Subtract/2
  Subtract/1 -> Gain8/1, Gain7/1
  PsiRef/1 -> Subtract1/1
  PsiEm/1 -> Subtract1/2
  Subtract1/1 -> ?  "PsiErr"

== system MotorCtrl_DTC_Math/HFTask/invParkTransform ==
  Ud : Inport
  Uq : Inport  Port=2
  SinTheta : Inport  Port=3
  CosTheta : Inport  Port=4
  Add : Sum
  Product{,1..3} (4 alike) : Product
  Subtract : Sum  Inputs=+-
  Ualpha : Outport
  Ubeta : Outport  Port=2
  wires:
  Uq/1 -> Product3/1, Product1/1
  Subtract/1 -> Ualpha/1  "Ualpha"
  CosTheta/1 -> Product/2, Product3/2
  SinTheta/1 -> Product2/2, Product1/2
  Product/1 -> Subtract/1
  Product1/1 -> Subtract/2
  Ud/1 -> Product/1, Product2/1
  Product2/1 -> Add/1
  Product3/1 -> Add/2
  Add/1 -> Ubeta/1  "Ubeta"

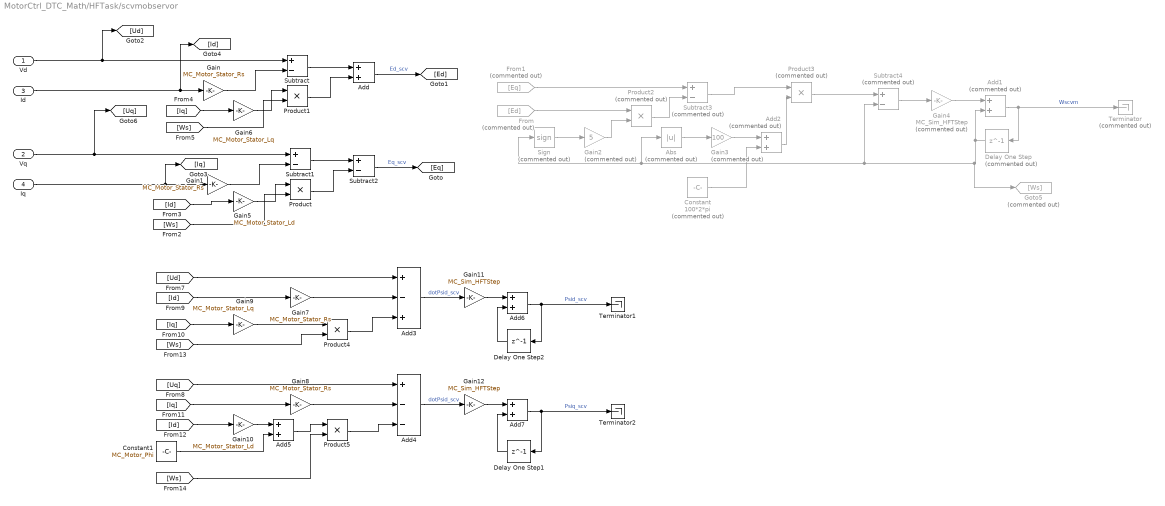
== system MotorCtrl_DTC_Math/HFTask/scvmobservor ==
  Vd : Inport
  Vq : Inport  Port=2
  Id : Inport  Port=3
  Iq : Inport  Port=4
  Abs : Abs  Commented=on  SaturateOnIntegerOverflow=off
  Add{,5..7} (4 alike) : Sum
  Add1 : Sum  Commented=on
  Add2 : Sum  Commented=on
  Add3 : Sum  Inputs=+-+
  Add4 : Sum  Inputs=+--
  Constant : Constant  Commented=on  Value=100*2*pi  OutDataTypeStr=single
  Constant1 : Constant  Value=MC_Motor_Phi  OutDataTypeStr=single
  Delay One Step : Delay  Commented=on  DelayLength=1
  Delay One Step1 : Delay  DelayLength=1
  Delay One Step2 : Delay  DelayLength=1
  From : From  Commented=on  GotoTag=Ed
  From1 : From  Commented=on  GotoTag=Eq
  Gain{,1,7..8} (4 alike) : Gain  Gain=MC_Motor_Stator_Rs
  Gain10 : Gain  Gain=MC_Motor_Stator_Ld
  Gain11 : Gain  Gain=MC_Sim_HFTStep
  Gain12 : Gain  Gain=MC_Sim_HFTStep
  Gain2 : Gain  Commented=on  Gain=5
  Gain3 : Gain  Commented=on  Gain=100
  Gain4 : Gain  Commented=on  Gain=MC_Sim_HFTStep
  Gain5 : Gain  Gain=MC_Motor_Stator_Ld
  Gain6 : Gain  Gain=MC_Motor_Stator_Lq
  Gain9 : Gain  Gain=MC_Motor_Stator_Lq
  Goto5 : Goto  Commented=on  GotoTag=Ws
  Product{,1,4..5} (4 alike) : Product
  Product2 : Product  Commented=on
  Product3 : Product  Commented=on
  Sign : Signum  Commented=on
  Subtract : Sum  Inputs=+-
  Subtract1 : Sum  Inputs=+-
  Subtract2 : Sum  Inputs=+-
  Subtract3 : Sum  Commented=on  Inputs=+-
  Subtract4 : Sum  Commented=on  Inputs=+-
  Terminator : Terminator  Commented=on
  Terminator1 : Terminator
  Terminator2 : Terminator
  wires:
  Product/1 -> Subtract2/2
  From1/1 -> Subtract3/1
  Gain11/1 -> Add6/1
  Add4/1 -> Gain12/1  "dotPsid_scv"
  Add5/1 -> Product5/1
  Gain8/1 -> Add4/2
  [Id] -> Gain5/1
  Add/1 -> [Ed]  "Ed_scv"
  Delay One Step2/1 -> Add6/2
  Add6/1 -> Terminator1/1, Delay One Step2/1  "Psid_scv"
  Product5/1 -> Add4/3
  [Ws] -> Product1/2
  [Ud] -> Add3/1
  Gain12/1 -> Add7/1
  Gain4/1 -> Add1/1
  Gain10/1 -> Add5/1
  [Iq] -> Gain6/1
  Delay One Step1/1 -> Add7/2
  Add3/1 -> Gain11/1  "dotPsid_scv"
  [Ws] -> Product4/2
  Abs/1 -> Gain3/1
  Gain3/1 -> Add2/1
  Subtract3/1 -> Product3/1
  [Uq] -> Add4/1
  [Id] -> Gain10/1
  Id/1 -> [Id], Gain/1
  Add2/1 -> Product3/2
  Gain9/1 -> Product4/1
  Gain2/1 -> Product2/2
  Constant/1 -> Add2/2
  Vd/1 -> Subtract/1, [Ud]
  Subtract1/1 -> Subtract2/1
  Delay One Step/1 -> Goto5/1, Subtract4/2, Abs/1, Sign/1, Add1/2
  Iq/1 -> [Iq], Gain1/1
  [Ws] -> Product5/2
  [Iq] -> Gain8/1
  Product1/1 -> Add/2
  Gain5/1 -> Product/1
  Product3/1 -> Subtract4/1
  Subtract4/1 -> Gain4/1
  Add1/1 -> Delay One Step/1, Terminator/1  "Wscvm"
  Gain7/1 -> Add3/2
  Add7/1 -> Terminator2/1, Delay One Step1/1  "Psiq_scv"
  Product2/1 -> Subtract3/2
  [Ws] -> Product/2
  Gain1/1 -> Subtract1/2
  Gain6/1 -> Product1/1
  From/1 -> Product2/1
  Product4/1 -> Add3/3
  Gain/1 -> Subtract/2
  Sign/1 -> Gain2/1
  [Iq] -> Gain9/1
  Subtract/1 -> Add/1
  Vq/1 -> [Uq], Subtract1/1
  [Id] -> Gain7/1
  Constant1/1 -> Add5/2
  Subtract2/1 -> [Eq]  "Eq_scv"

== system MotorCtrl_DTC_Math/HFTask/smo ==
  Valpha : Inport
  Vbeta : Inport  Port=2
  Ialpha : Inport  Port=3
  Ibeta : Inport  Port=4
  getE : Subsystem
  getSpeedandTheta : Subsystem
  Speed : Outport
  Theta : Outport  Port=2
  wires:
  Valpha/1 -> getE/1(Valpha)
  Vbeta/1 -> getE/2(Vbeta)
  Ialpha/1 -> getE/3(Ialpha)
  Ibeta/1 -> getE/4(Ibeta)
  getE/1(Ealpha) -> getSpeedandTheta/1(Ealpha)
  getE/2(Ebeta) -> getSpeedandTheta/2(Ebeta)
  getSpeedandTheta/1(Speed) -> Speed/1
  getSpeedandTheta/2(Theta) -> Theta/1

== system MotorCtrl_DTC_Math/HFTask/svpwm ==
  Valpha : Inport
  Vbeta : Inport  Port=2
  Vdc : Inport  Port=3
  Ia : Inport  Port=4
  Ib : Inport  Port=5
  PhaseShortEnableFlag : Inport  Port=6
  Terminator : Terminator
  getVoltageExchange : Subsystem
  setDTCompelte : Subsystem
  setPhaseandSample_ORS_Double : Subsystem
  DutySVPWM : Outport
  SamplePoint : Outport  Port=2
  SampleValid : Outport  Port=3
  SectorN : Outport  Port=4
  wires:
  Valpha/1 -> getVoltageExchange/1(Valpha)
  Vbeta/1 -> getVoltageExchange/2(Vbeta)
  Vdc/1 -> getVoltageExchange/3(Vdc)
  getVoltageExchange/1(Va) -> setDTCompelte/1(Va)
  getVoltageExchange/2(Vb) -> setDTCompelte/2(Vb)
  getVoltageExchange/3(Vc) -> setDTCompelte/3(Vc)
  getVoltageExchange/4(Vmed) -> setDTCompelte/4(Vmed)
  Ia/1 -> setDTCompelte/5(Ia)
  Ib/1 -> setDTCompelte/6(ib)
  setDTCompelte/1(SectorN) -> SectorN/1, setPhaseandSample_ORS_Double/1(SectorN)
  setDTCompelte/2(DutyLMS) -> setPhaseandSample_ORS_Double/2(DutyLMS)
  setPhaseandSample_ORS_Double/1(DutySVPWM) -> DutySVPWM/1
  setPhaseandSample_ORS_Double/2(SamplePoint) -> SamplePoint/1
  setPhaseandSample_ORS_Double/3(SampleValid) -> SampleValid/1
  PhaseShortEnableFlag/1 -> Terminator/1

== system MotorCtrl_DTC_Math/HFTask/voltageLimit ==
  UdRef : Inport
  UqRef : Inport  Port=2
  Umax : Inport  Port=3
  Add : Sum
  Compare To Constant : simulink/Logic and Bit Operations/Compare To Constant  relop=<=  const=0  OutDataTypeStr=boolean
  Compare To Constant1 : simulink/Logic and Bit Operations/Compare To Constant  relop=>=  const=0  OutDataTypeStr=boolean
  Constant : Constant  Value=0  OutDataTypeStr=single
  Gain : Gain  Gain=-1
  Gain1 : Gain  Gain=-1
  Product : Product
  Saturation Dynamic : simulink/Discontinuities/Saturation Dynamic  OutMin=[]  OutMax=[]  OutDataTypeStr=Inherit: Same as second input  OutDataType=fixdt(1, 16)  OutScaling=2^-10  DoSatur=off
  Sqrt : Sqrt
  Subtract : Sum  Inputs=+-
  Switch : Switch  Criteria=u2 > Threshold  SaturateOnIntegerOverflow=off  InputSameDT=off
  Switch1 : Switch  Criteria=u2 > Threshold  SaturateOnIntegerOverflow=off  InputSameDT=off
  Switch2 : Switch  Criteria=u2 > Threshold  SaturateOnIntegerOverflow=off  InputSameDT=off
  Ud : Outport
  Uq : Outport  Port=2
  wires:
  Add/1 -> Product/1
  Subtract/1 -> Product/2
  Product/1 -> Compare To Constant/1, Sqrt/1
  Compare To Constant/1 -> [UdOverFlow]
  Sqrt/1 -> Gain/1, Saturation Dynamic/1
  Gain/1 -> Saturation Dynamic/3
  UdRef/1 -> [UdRef]
  UqRef/1 -> [UqRef]
  Umax/1 -> [Umax]
  [Umax] -> Subtract/1, Add/1
  [UdRef] -> Add/2, Subtract/2
  [UqRef] -> Saturation Dynamic/2
  Saturation Dynamic/1 -> Switch/3
  [UdOverFlow] -> Switch/2
  Constant/1 -> Switch/1
  Switch/1 -> Uq/1  "UqLimit"
  Switch1/1 -> Ud/1  "UdLimit"
  Switch2/1 -> Switch1/1
  [UdRef] -> Compare To Constant1/1
  Compare To Constant1/1 -> Switch2/2
  [Umax] -> Gain1/1, Switch2/1
  Gain1/1 -> Switch2/3
  [UdOverFlow] -> Switch1/2
  [UdRef] -> Switch1/3

== system MotorCtrl_DTC_Math/Hardware_Math/AngleProcess ==
  In1 : Inport
  Constant : Constant  Value=2*pi  SampleTime=-1
  Data Type Conversion : DataTypeConversion  OutDataTypeStr=single  SaturateOnIntegerOverflow=off  RndMeth=Floor
  Mod : Math  Operator=mod
  Out1 : Outport
  wires:
  Mod/1 -> Data Type Conversion/1
  In1/1 -> Mod/1
  Constant/1 -> Mod/2
  Data Type Conversion/1 -> Out1/1  "ThetaM"
